simulink model "dom3_sim"  (R2014a)
settings: Solver=ode45  StartTime=0.0  StopTime=300000  RelTol=1e-3
values from neighbouring files (symbols this model uses):
  Cpw = 4190    [blok.m]    (also in dom.m)
  Cvg = Cpw*Rw*Vw    (= 838000)    [blok.m]    (also in dom.m = 628500000)
  Cvk = Cpp*Rw*Vk    (= 201000)    [blok.m]    (also in dom.m = 2010000)
  Cvw = (Cvw1+Cvs)/2    [blok.m]    (also in dom.m = 2347.68)
  dfk1 = 0    [blok.m]
  dfk2 = 0    [blok.m]
  dTwew = 0    [blok.m]
  dTwew1 = 2    [blok.m]
  dTwew2 = 0    [blok.m]
  dTzew = 0    [blok.m]    (also in dom.m)
  fk10 = fmg1/Rw    (= 5.42417010197e-05)    [blok.m]
  fk20 = fmg2/Rw    (= 6.50900412237e-05)    [blok.m]
  Kcg1 = qg1/(TkpN-Twew1N)    (= 90.9090909091)    [blok.m]
  Kcg2 = qg2/(TkpN-Twew2N)    (= 109.090909091)    [blok.m]
  Kcs = Kcw1*(pp/ps)/2    [blok.m]
  Kcw1 = qg1/(Twew1N-TzewN)    (= 113.636363636)    [blok.m]
  Kcw2 = qg2/(Twew2N-TzewN)    (= 136.363636364)    [blok.m]
  q1 = 0    [blok.m]
  q2 = 0    [blok.m]
  Rw = 1000    [blok.m]    (also in dom.m)
  Tgp10 = x(2,1)    [blok.m]
  Tgp20 = x(4,1)    [blok.m]
  Tkz0 = x(5,1)    [blok.m]    (also in dom.m = 90)
  ts = 1000    [blok.m]
  Twew10 = x(1,1)    [blok.m]
  Twew20 = x(3,1)    [blok.m]
  Tzew0 = TzewN    (= -20)    [blok.m]    (also in dom.m)
undefined symbols (not defined in the file): qk0, qkN, ZI, ZP
settings Model: Creator=Adrian  LastModifiedBy=Adrian

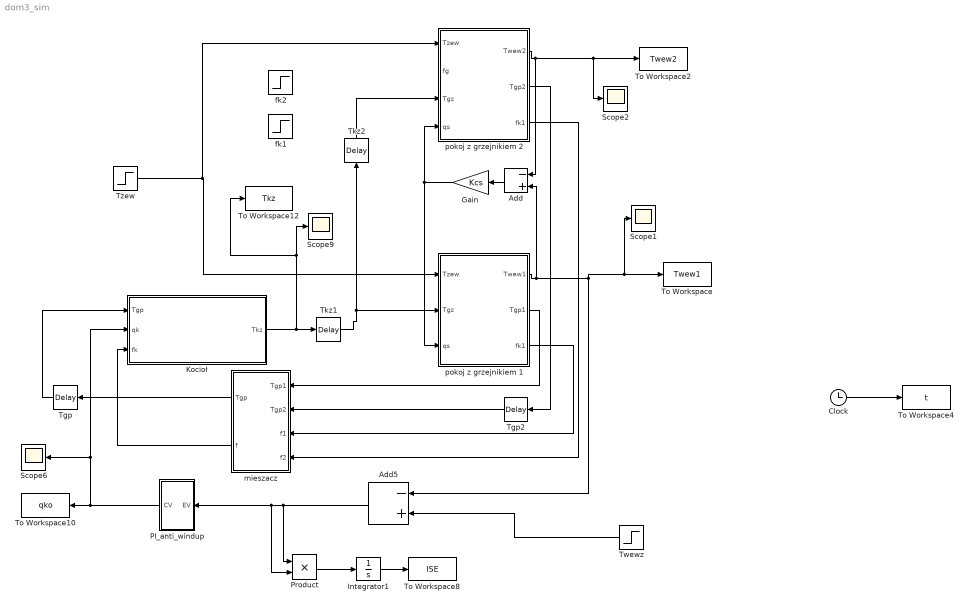
== system dom3_sim ==
  Add : Sum  Inputs=-+
  Add5 : Sum  Inputs=-+
  Clock : Clock
  Gain : Gain  Gain=Kcs
  Integrator1 : Integrator
  Kocioł : Subsystem  mask{Cpw=Cpw, Rw=Rw, Cvk=Cvk, Tz0=Tkz0}
      mask prompts: Tz0 "Tkz0"
  PI_anti_windup : Subsystem  mask{Kp=ZP, Ki=ZI, WP=qk0, Ka=10, Lim=qkN*10}
  Product : Product
  Scope{1..2,6,9} (4 alike) : Scope
      Scope1 settings: TimeRange=20000000  YMin=19  YMax=21.5
      Scope2 settings: TimeRange=20000000  YMin=19  YMax=21.5
      Scope6 settings: TimeRange=20000000  YMin=19  YMax=21.5  SaveName=ScopeData6
      Scope9 settings: TimeRange=400000  YMin=17.5  YMax=20  SaveName=ScopeData10
  Tgp : TransportDelay  DelayTime=300  InitialOutput=(Tgp10*fk10+Tgp20*fk20)/(fk10+fk20)
  Tgp2 : TransportDelay  DelayTime=300  InitialOutput=Tgp20
  Tkz1 : TransportDelay  DelayTime=300  InitialOutput=Tkz0
  Tkz2 : TransportDelay  DelayTime=300  InitialOutput=Tkz0
  To Workspace : ToWorkspace  VariableName=Twew1  SampleTime=-1
  To Workspace10 : ToWorkspace  VariableName=qko  SampleTime=-1
  To Workspace12 : ToWorkspace  VariableName=Tkz  SampleTime=-1
  To Workspace2 : ToWorkspace  VariableName=Twew2  SampleTime=-1
  To Workspace4 : ToWorkspace  VariableName=t  SampleTime=-1
  To Workspace8 : ToWorkspace  VariableName=ISE  SampleTime=-1
  Twewz : Step  Time=ts  Before=Twew10  After=Twew10+dTwew  SampleTime=0
  "Tzew " : Step  Time=ts  Before=Tzew0  After=Tzew0+dTzew  SampleTime=0
  fk1 : Step  Time=ts  Before=fk10  After=fk10+dfk1  SampleTime=0
  fk2 : Step  Time=ts  Before=fk20  After=fk20+dfk2  SampleTime=0
  mieszacz : Subsystem
  pokoj z grzejnikiem 2 : Subsystem  mask{Kcg=Kcg2, Kcw=Kcw2, Cvw=Cvw, Cvg=Cvg, Twew0=Twew20, Tgp0=Tgp20, Cpw=Cpw, Rw=Rw}
  "pokoj z grzejnikiem 1 " : Subsystem  mask{Kcg=Kcg1, Kcw=Kcw1, Cvw=Cvw, Cvg=Cvg, Twew0=Twew10, Tgp0=Tgp10, Cpw=Cpw, Rw=Rw}
  wires:
  "Tzew "/1 -> pokoj z grzejnikiem 2/1(Tzew), "pokoj z grzejnikiem 1 "/1(Tzew)
  "pokoj z grzejnikiem 1 "/1(Twew1) -> Add/2, Add5/1, Scope1/1, To Workspace/1
  pokoj z grzejnikiem 2/1(Twew2) -> Add/1, Scope2/1, To Workspace2/1
  mieszacz/2(f) -> Kocioł/3(fk)
  Add/1 -> Gain/1
  Gain/1 -> "pokoj z grzejnikiem 1 "/3(qs), pokoj z grzejnikiem 2/4(qs)
  Kocioł/1(Tkz) -> To Workspace12/1, Scope9/1, Tkz1/1
  "pokoj z grzejnikiem 1 "/2(Tgp1) -> mieszacz/1(Tgp1)
  Tgp2/1 -> mieszacz/2(Tgp2)
  pokoj z grzejnikiem 2/2(Tgp2) -> Tgp2/1
  Tkz2/1 -> pokoj z grzejnikiem 2/3(Tgz)
  Tkz1/1 -> "pokoj z grzejnikiem 1 "/2(Tgz), Tkz2/1
  mieszacz/1(Tgp) -> Tgp/1
  Tgp/1 -> Kocioł/1(Tgp)
  Clock/1 -> To Workspace4/1
  Product/1 -> Integrator1/1
  Integrator1/1 -> To Workspace8/1
  PI_anti_windup/1(CV) -> To Workspace10/1, Kocioł/2(qk), Scope6/1
  Add5/1 -> Product/1, Product/2, PI_anti_windup/1(EV)
  Twewz/1 -> Add5/2
  "pokoj z grzejnikiem 1 "/3(fk1) -> mieszacz/3(f1)
  pokoj z grzejnikiem 2/3(fk1) -> mieszacz/4(f2)

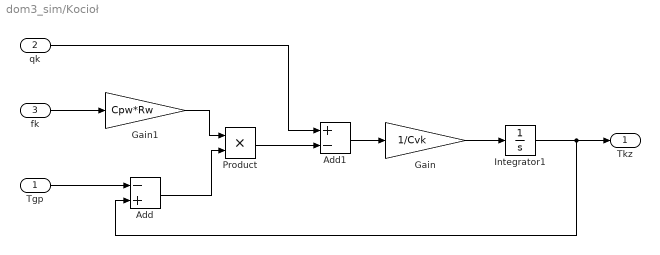
== system dom3_sim/Kocioł ==
  Tgp : Inport
  qk : Inport  Port=2
  fk : Inport  Port=3
  Add : Sum  Inputs=-+
  Add1 : Sum  Inputs=+-
  Gain : Gain  Gain=1/Cvk
  Gain1 : Gain  Gain=Cpw*Rw
  Integrator1 : Integrator  InitialCondition=Tkz0
  Product : Product
  Tkz : Outport
  wires:
  Gain/1 -> Integrator1/1
  Integrator1/1 -> Add/2, Tkz/1
  Tgp/1 -> Add/1
  fk/1 -> Gain1/1
  Gain1/1 -> Product/1
  Add/1 -> Product/2
  qk/1 -> Add1/1
  Product/1 -> Add1/2
  Add1/1 -> Gain/1

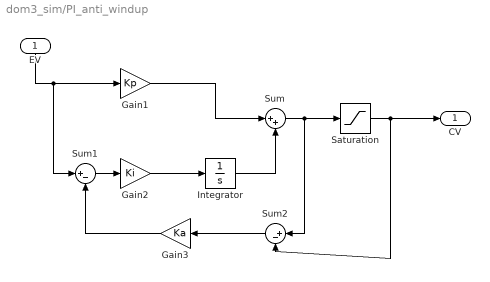
== system dom3_sim/PI_anti_windup ==
  EV : Inport
  Gain1 : Gain  Gain=Kp
  Gain2 : Gain  Gain=Ki
  Gain3 : Gain  Gain=Ka
  Integrator : Integrator  InitialCondition=WP
  Saturation : Saturate  UpperLimit=Lim
  Sum : Sum  Inputs=|++
  Sum1 : Sum  Inputs=|+-
  Sum2 : Sum  Inputs=|+-
  CV : Outport
  wires:
  Gain2/1 -> Integrator/1
  Integrator/1 -> Sum/2
  EV/1 -> Sum1/1, Gain1/1
  Gain1/1 -> Sum/1
  Sum1/1 -> Gain2/1
  Gain3/1 -> Sum1/2
  Sum2/1 -> Gain3/1
  Saturation/1 -> Sum2/2, CV/1
  Sum/1 -> Sum2/1, Saturation/1

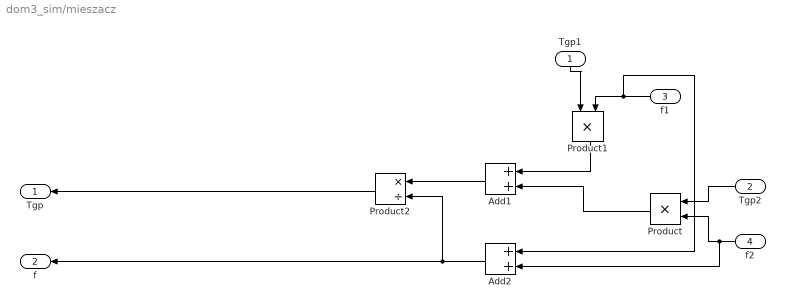
== system dom3_sim/mieszacz ==
  Tgp1 : Inport
  Tgp2 : Inport  Port=2
  f1 : Inport  Port=3
  f2 : Inport  Port=4
  Add1 : Sum
  Add2 : Sum
  Product : Product
  Product1 : Product
  Product2 : Product  Inputs=*/
  Tgp : Outport
  f : Outport  Port=2
  wires:
  Product2/1 -> Tgp/1
  Add1/1 -> Product2/1
  Tgp2/1 -> Product/1
  f2/1 -> Add2/2, Product/2
  Tgp1/1 -> Product1/1
  f1/1 -> Add2/1, Product1/2
  Product1/1 -> Add1/1
  Product/1 -> Add1/2
  Add2/1 -> Product2/2, f/1

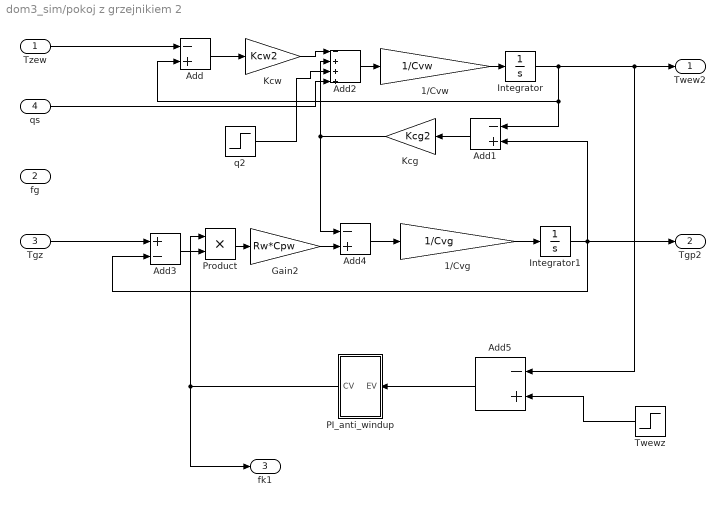
== system dom3_sim/pokoj z grzejnikiem 2 ==
  Tzew : Inport
  fg : Inport  Port=2
  Tgz : Inport  Port=3
  qs : Inport  Port=4
  1/Cvg : Gain  Gain=1/Cvg
  1/Cvw : Gain  Gain=1/Cvw
  Add{,1,4..5} (4 alike) : Sum  Inputs=-+
  Add2 : Sum  Inputs=-+++
  Add3 : Sum  Inputs=+-
  Gain2 : Gain  Gain=Rw*Cpw
  Integrator : Integrator  InitialCondition=Twew20
  Integrator1 : Integrator  InitialCondition=Tgp20
  "Kcg " : Gain  Gain=Kcg2
  Kcw : Gain  Gain=Kcw2
  PI_anti_windup : Subsystem  mask{Kp=ZP, Ki=ZI, WP=fk20, Ka=10, Lim=fk20*1}
  Product : Product
  Twewz : Step  Time=ts  Before=Twew10  After=Twew10+dTwew2  SampleTime=0
  q2 : Step  Time=ts  After=q2  SampleTime=0
  Twew2 : Outport
  Tgp2 : Outport  Port=2
  fk1 : Outport  Port=3
  wires:
  Kcw/1 -> Add2/1
  1/Cvg/1 -> Integrator1/1
  "Kcg "/1 -> Add4/1, Add2/2
  Add/1 -> Kcw/1
  Add2/1 -> 1/Cvw/1
  1/Cvw/1 -> Integrator/1
  Tzew/1 -> Add/1
  Add4/1 -> 1/Cvg/1
  Gain2/1 -> Add4/2
  Add3/1 -> Product/2
  Tgz/1 -> Add3/1
  Product/1 -> Gain2/1
  Add1/1 -> "Kcg "/1
  Integrator1/1 -> Tgp2/1, Add1/2, Add3/2
  q2/1 -> Add2/3
  qs/1 -> Add2/4
  Integrator/1 -> Add1/1, Add/2, Add5/1, Twew2/1
  Twewz/1 -> Add5/2
  Add5/1 -> PI_anti_windup/1(EV)
  PI_anti_windup/1(CV) -> Product/1, fk1/1

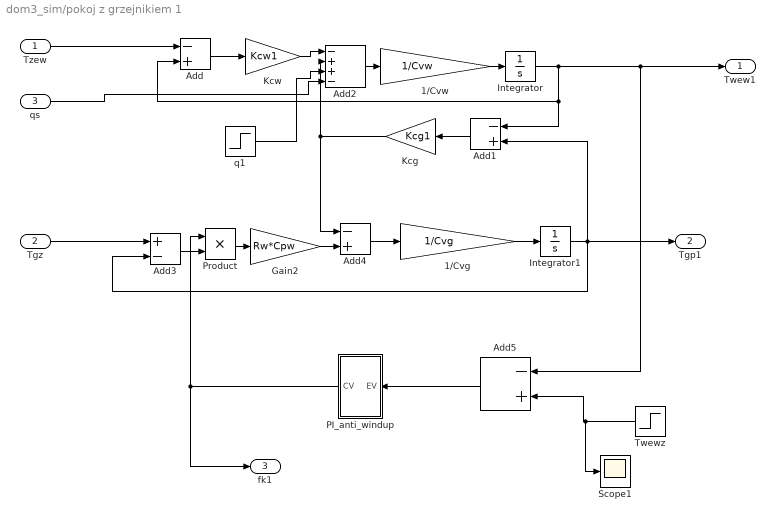
== system dom3_sim/pokoj z grzejnikiem 1  ==
  Tzew : Inport
  Tgz : Inport  Port=2
  qs : Inport  Port=3
  1/Cvg : Gain  Gain=1/Cvg
  1/Cvw : Gain  Gain=1/Cvw
  Add{,1,4..5} (4 alike) : Sum  Inputs=-+
  Add2 : Sum  Inputs=-++-
  Add3 : Sum  Inputs=+-
  Gain2 : Gain  Gain=Rw*Cpw
  Integrator : Integrator  InitialCondition=Twew10
  Integrator1 : Integrator  InitialCondition=Tgp10
  "Kcg " : Gain  Gain=Kcg1
  Kcw : Gain  Gain=Kcw1
  PI_anti_windup : Subsystem  mask{Kp=ZP, Ki=ZI, WP=fk10, Ka=10, Lim=fk10*1}
  Product : Product
  Scope1 : Scope
      settings: TimeRange=20000000  YMin=19  YMax=21.5  SaveName=ScopeData2
  Twewz : Step  Time=ts  Before=Twew10  After=Twew10+dTwew1  SampleTime=0
  q1 : Step  Time=ts  After=q1  SampleTime=0
  Twew1 : Outport
  Tgp1 : Outport  Port=2
  fk1 : Outport  Port=3
  wires:
  Kcw/1 -> Add2/1
  1/Cvg/1 -> Integrator1/1
  "Kcg "/1 -> Add4/1, Add2/2
  Add/1 -> Kcw/1
  Add2/1 -> 1/Cvw/1
  1/Cvw/1 -> Integrator/1
  Tzew/1 -> Add/1
  Add4/1 -> 1/Cvg/1
  Gain2/1 -> Add4/2
  Add3/1 -> Product/2
  Tgz/1 -> Add3/1
  Product/1 -> Gain2/1
  Add1/1 -> "Kcg "/1
  Integrator1/1 -> Tgp1/1, Add1/2, Add3/2
  Integrator/1 -> Add1/1, Add/2, Add5/1, Twew1/1
  q1/1 -> Add2/3
  qs/1 -> Add2/4
  Twewz/1 -> Scope1/1, Add5/2
  Add5/1 -> PI_anti_windup/1(EV)
  PI_anti_windup/1(CV) -> Product/1, fk1/1

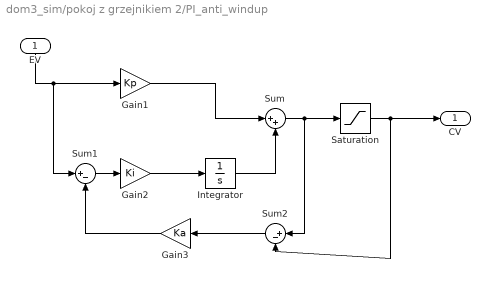
== system dom3_sim/pokoj z grzejnikiem 2/PI_anti_windup ==
  EV : Inport
  Gain1 : Gain  Gain=Kp
  Gain2 : Gain  Gain=Ki
  Gain3 : Gain  Gain=Ka
  Integrator : Integrator  InitialCondition=WP
  Saturation : Saturate  UpperLimit=Lim
  Sum : Sum  Inputs=|++
  Sum1 : Sum  Inputs=|+-
  Sum2 : Sum  Inputs=|+-
  CV : Outport
  wires:
  Gain2/1 -> Integrator/1
  Integrator/1 -> Sum/2
  EV/1 -> Sum1/1, Gain1/1
  Gain1/1 -> Sum/1
  Sum1/1 -> Gain2/1
  Gain3/1 -> Sum1/2
  Sum2/1 -> Gain3/1
  Saturation/1 -> Sum2/2, CV/1
  Sum/1 -> Sum2/1, Saturation/1

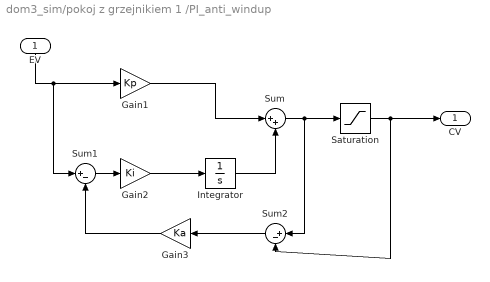
== system dom3_sim/pokoj z grzejnikiem 1 /PI_anti_windup ==
  EV : Inport
  Gain1 : Gain  Gain=Kp
  Gain2 : Gain  Gain=Ki
  Gain3 : Gain  Gain=Ka
  Integrator : Integrator  InitialCondition=WP
  Saturation : Saturate  UpperLimit=Lim
  Sum : Sum  Inputs=|++
  Sum1 : Sum  Inputs=|+-
  Sum2 : Sum  Inputs=|+-
  CV : Outport
  wires:
  Gain2/1 -> Integrator/1
  Integrator/1 -> Sum/2
  EV/1 -> Sum1/1, Gain1/1
  Gain1/1 -> Sum/1
  Sum1/1 -> Gain2/1
  Gain3/1 -> Sum1/2
  Sum2/1 -> Gain3/1
  Saturation/1 -> Sum2/2, CV/1
  Sum/1 -> Sum2/1, Saturation/1
